simulink model "simulacija_pejsmejker"  (R2018a)
settings: Solver=VariableStepAuto  StartTime=0.0  StopTime=10  RelTol=1e-3
values from neighbouring files (symbols this model uses):
  B = 5.28    [racun_ki.m]    (also in z1_3.m)
  k = 2.64    [racun_ki.m]    (also in z1_3.m)
  ki = prvi_clan/drugi_clan    (= 1.96883116883)    [racun_ki.m]    (also in z1_3.m = 5)
  ki2 = 0.833 * T_u    (= 0.4165)    [z1_3.m]
  kp = 153    [racun_ki.m]    (also in z1_3.m = 12)
  kp2 = 0.45 * K_u    (= 68.99832)    [z1_3.m]
  M = 0.264    [racun_ki.m]    (also in z1_3.m)
  T = 0.001    [z1_3.m]
settings Model: Creator=djoco  LastModifiedBy=djoco

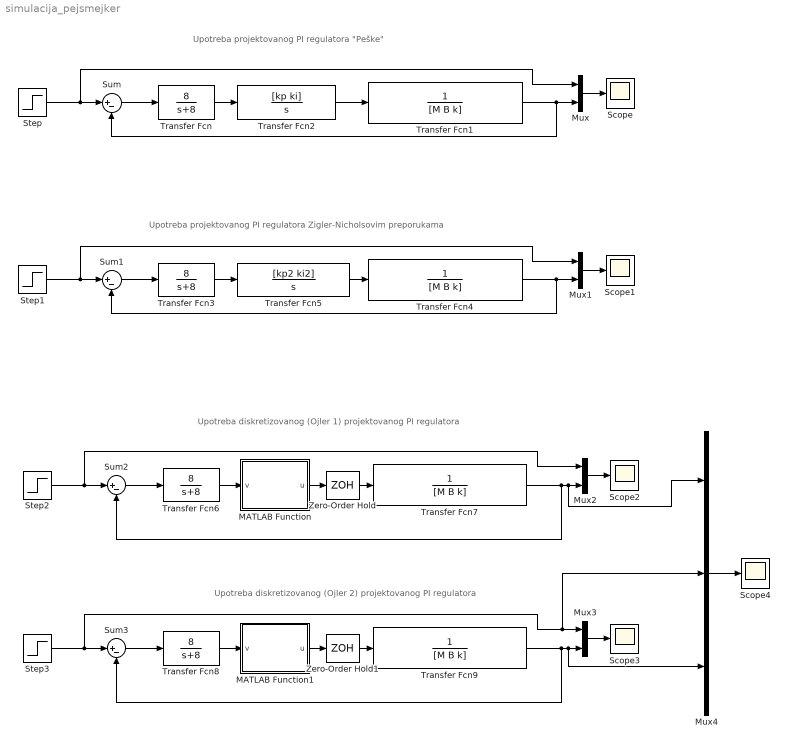
== system simulacija_pejsmejker ==
  note: Upotreba projektovanog PI regulatora "Peške"
  note: Upotreba projektovanog PI regulatora Zigler-Nicholsovim preporukama
  note: Upotreba diskretizovanog (Ojler 1) projektovanog PI regulatora
  note: Upotreba diskretizovanog (Ojler 2) projektovanog PI regulatora
  MATLAB Function : MATLAB Function  TreatAsAtomicUnit=on
  MATLAB Function1 : MATLAB Function  TreatAsAtomicUnit=on
  Mux{,1..3} (4 alike) : Mux  Inputs=2
  Mux4 : Mux  Inputs=3
  Scope{,1..4} (5 alike) : Scope
  Step{,1..3} (4 alike) : Step  After=70  SampleTime=0
  Sum{,1..3} (4 alike) : Sum  Inputs=|+-
  Transfer Fcn{,3,6,8} (4 alike) : TransferFcn  Numerator=[8]  Denominator=[1 8]
  Transfer Fcn{1,4,7,9} (4 alike) : TransferFcn  Denominator=[M B k]
  Transfer Fcn2 : TransferFcn  Numerator=[kp ki]  Denominator=[1 0]
  Transfer Fcn5 : TransferFcn  Numerator=[kp2 ki2]  Denominator=[1 0]
  Zero-Order Hold : ZeroOrderHold  SampleTime=-1
  Zero-Order Hold1 : ZeroOrderHold  SampleTime=-1
  wires:
  Transfer Fcn1/1 -> Mux/2, Sum/2
  Sum/1 -> Transfer Fcn/1
  Step/1 -> Mux/1, Sum/1
  Mux/1 -> Scope/1
  Transfer Fcn/1 -> Transfer Fcn2/1
  Transfer Fcn2/1 -> Transfer Fcn1/1
  Sum1/1 -> Transfer Fcn3/1
  Transfer Fcn5/1 -> Transfer Fcn4/1
  Step1/1 -> Mux1/1, Sum1/1
  Transfer Fcn3/1 -> Transfer Fcn5/1
  Transfer Fcn4/1 -> Mux1/2, Sum1/2
  Mux1/1 -> Scope1/1
  Mux2/1 -> Scope2/1
  Step2/1 -> Mux2/1, Sum2/1
  Sum2/1 -> Transfer Fcn6/1
  Transfer Fcn7/1 -> Mux4/1, Mux2/2, Sum2/2
  Transfer Fcn6/1 -> MATLAB Function/1(v)
  MATLAB Function/1(u) -> Zero-Order Hold/1
  Zero-Order Hold/1 -> Transfer Fcn7/1
  Transfer Fcn8/1 -> MATLAB Function1/1(v)
  Transfer Fcn9/1 -> Mux4/3, Mux3/2, Sum3/2
  Zero-Order Hold1/1 -> Transfer Fcn9/1
  MATLAB Function1/1(u) -> Zero-Order Hold1/1
  Sum3/1 -> Transfer Fcn8/1
  Mux3/1 -> Scope3/1
  Step3/1 -> Mux4/2, Mux3/1, Sum3/1
  Mux4/1 -> Scope4/1

== matlab function simulacija_pejsmejker/MATLAB Function1 ==
  settings: updateMethod=DISCRETE
  data: v input; u output; kp parameter; ki parameter; T parameter
function u  = ojler2_PI(v, kp, ki, T)

persistent Ip

if isempty(Ip)
    Ip = 0;
end

P = kp*v;
I = Ip + ki*T*v;

u = P + I;

Ip = I;

== matlab function simulacija_pejsmejker/MATLAB Function ==
  settings: updateMethod=DISCRETE
  data: v input; u output; kp parameter; ki parameter; T parameter
function u  = ojler1_PI(v, kp, ki, T)

persistent Ip  vp

if isempty(Ip)
    Ip = 0;
end

if isempty(vp)
    vp = 0;
end

P = kp*v;
I = Ip + ki*T*vp;

u = P + I;

vp = v;
Ip = I;
